simulink model "missile"  (Simulink 8.6)
settings: Solver=ode3  StartTime=0.0  StopTime=60  FixedStep=0.01  RelTol=1e-3
settings Model: Creator=½¯·æ  LastModifiedBy=Administrator
settings DataIOCC: LimitDataPoints=off
settings DebuggingCC: FcnCallInpInsideContextMsg=UseLocalSettings  InitInArrayFormatMsg=none

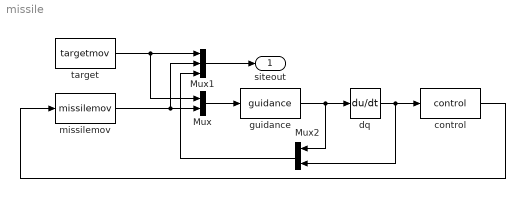
== system missile ==
  Mux : Mux  Inputs=2
  Mux1 : Mux  Inputs=3
  Mux2 : Mux  Inputs=2
  control : MATLABFcn  MATLABFcn=control
  dq : Derivative
  guidance : MATLABFcn  MATLABFcn=guidance
  missilemov : S-Function  FunctionName=missilemov  SFunctionDeploymentMode=off  EnableBusSupport=off
  target : S-Function  FunctionName=targetmov  SFunctionDeploymentMode=off  EnableBusSupport=off
  siteout : Outport
  wires:
  Mux/1 -> guidance/1
  target/1 -> Mux/1, Mux1/1
  missilemov/1 -> Mux/2, Mux1/2
  dq/1 -> control/1, Mux2/2
  control/1 -> missilemov/1
  guidance/1 -> dq/1, Mux2/1
  Mux1/1 -> siteout/1
  Mux2/1 -> Mux1/3
